simulink model "DC_motor_simulink_PID_like_fuzzy"  (R2019a)
settings: Solver=VariableStepAuto  StartTime=0.0  StopTime=10.0  RelTol=1e-3
values from neighbouring files (symbols this model uses):
  A = [-b/J K/J; -K/L -R/L]    [dc_motor_speed_PID_like_fuzzy_control.m]
  B = [0; 1/L]    [dc_motor_speed_PID_like_fuzzy_control.m]
  C = [0 1]    [dc_motor_speed_PID_like_fuzzy_control.m]
  D = [0]    [dc_motor_speed_PID_like_fuzzy_control.m]
libraries: fuzblock x1
settings Model: Creator=ADHM  LastModifiedBy=ADHM

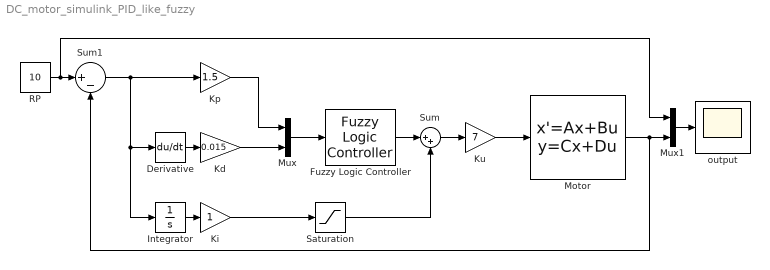
== system DC_motor_simulink_PID_like_fuzzy ==
  Derivative : Derivative
  Fuzzy Logic Controller : fuzblock/Fuzzy Logic  Controller  FIS='DC_motor.fis'  OutputSampleNumber=101  DataType=double  FuzzifiedInputs=off  RuleFiringStrengths=off  RuleOutputs=off  AggregatedOutputs=off  SimulateUsing=Interpreted execution  OutOfRangeInputValueMessage=warning  NoRuleFiredMessage=warning  EmptyOutputFuzzySetMessage=warning
  Integrator : Integrator
  Kd : Gain  Gain=0.015
  Ki : Gain
  Kp : Gain  Gain=1.5
  Ku : Gain  Gain=7
  Motor : StateSpace  A=A  B=B  C=C  D=D  InitialCondition=0
  Mux : Mux  Inputs=2
  Mux1 : Mux  Inputs=2
  RP : Constant  Value=10
  Saturation : Saturate  UpperLimit=1.5  LowerLimit=-1.5
  Sum : Sum  Inputs=|++
  Sum1 : Sum  Inputs=|+-
  output : Scope
  wires:
  Kp/1 -> Mux/1
  Kd/1 -> Mux/2
  Fuzzy Logic Controller/1 -> Sum/1
  Sum/1 -> Ku/1
  Ki/1 -> Saturation/1
  Ku/1 -> Motor/1
  Mux/1 -> Fuzzy Logic Controller/1
  RP/1 -> Mux1/1, Sum1/1
  Motor/1 -> Sum1/2, Mux1/2
  Derivative/1 -> Kd/1
  Sum1/1 -> Kp/1, Integrator/1, Derivative/1
  Integrator/1 -> Ki/1
  Mux1/1 -> output/1
  Saturation/1 -> Sum/2
